simulink model "birotorPVTOL"  (Simulink 7.5)
settings: Solver=ode45  StartTime=0.0  StopTime=10  RelTol=1e-3
values from neighbouring files (symbols this model uses):
  x0 = input('Introduzca x0: ')    [practicaCuadriRotor.m]    (also in practicaPVTOL.m)
  xf = input('Introduzca xf: ')    [practicaCuadriRotor.m]    (also in practicaPVTOL.m)
  y0 = input('Introduzca y0: ')    [practicaCuadriRotor.m]    (also in practicaPVTOL.m)
  yf = input('Introduzca yf: ')    [practicaCuadriRotor.m]    (also in practicaPVTOL.m)
settings Model: Creator=Celeste Anaid  LastModifiedBy=Mariano
settings OptimizationCC: ExpressionDepthLimit=128
settings DebuggingCC: MultiTaskDSMMsg=warning  MultiTaskCondExecSysMsg=none  FcnCallInpInsideContextMsg=Enable All  StrictBusMsg=None
settings RTWCC: IncludeERTFirstTime=on
settings CodeAppCC: CustomSymbolStrType=$N$R$M_T
settings GRTTargetCC: CombineOutputUpdateFcns=on

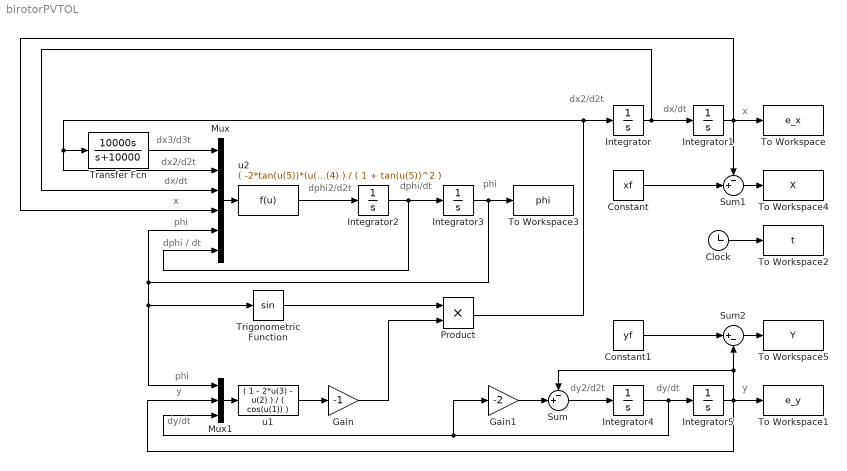
== system birotorPVTOL ==
  note: dy/dt
  note: y
  note: phi
  note: dy/dt
  note: dy2/d2t
  note: phi
  note: dphi/dt
  note: dphi2/d2t
  note: phi
  note: dphi / dt
  note: x
  note: dx/dt
  note: dx3/d3t
  note: dx2/d2t
  note: x
  note: dx/dt
  note: dx2/d2t
  note: y
  Clock : Clock
      settings: Decimation=10
  Constant : Constant  Value=xf  OutDataType=fixdt(1, 16)  OutScaling=2^0
  Constant1 : Constant  Value=yf  OutDataType=fixdt(1, 16)  OutScaling=2^0
  Gain : Gain  Gain=-1
  Gain1 : Gain  Gain=-2
  Integrator{,2..4} (4 alike) : Integrator
  Integrator1 : Integrator  InitialCondition=xf-x0
  Integrator5 : Integrator  InitialCondition=yf-y0
  Mux : Mux  Inputs=6
  Mux1 : Mux  Inputs=3
  Product : Product
  Sum : Sum  Inputs=-+|
  Sum1 : Sum  Inputs=-+|  OutDataType=fixdt(1, 16)  OutScaling=2^0
  Sum2 : Sum  Inputs=|+-  OutDataType=fixdt(1, 16)  OutScaling=2^0
  To Workspace : ToWorkspace  VariableName=e_x  SampleTime=-1  SaveFormat=Array
  To Workspace1 : ToWorkspace  VariableName=e_y  SampleTime=-1  SaveFormat=Array
  To Workspace2 : ToWorkspace  VariableName=t  SampleTime=-1  SaveFormat=Array
  To Workspace3 : ToWorkspace  VariableName=phi  SampleTime=-1  SaveFormat=Array
  To Workspace4 : ToWorkspace  VariableName=X  SampleTime=-1  SaveFormat=Array
  To Workspace5 : ToWorkspace  VariableName=Y  SampleTime=-1  SaveFormat=Array
  Transfer Fcn : TransferFcn  Numerator=[10000 0]  Denominator=[1 10000]
  Trigonometric Function : Trigonometry
  u1 : Fcn  Expr=( 1 - 2*u(3) - u(2) ) / ( cos(u(1)) )
  u2 : Fcn  Expr=|
      | ( -2*tan(u(5))*(u(6)^2)*(1+tan(u(5))^2)
      | -2*(1+tan(u(5))^2)*u(6) -tan(u(5)) +2*u(1) +5*u(2) +4*u(3) + u(4) ) / ( 1 + tan(u(5))^2 )
  wires:
  Transfer Fcn/1 -> Mux/1
  Integrator/1 -> Mux/3, Integrator1/1
  Integrator1/1 -> Mux/4, To Workspace/1, Sum1/1
  Mux/1 -> u2/1
  u2/1 -> Integrator2/1
  Integrator2/1 -> Integrator3/1, Mux/6
  Integrator3/1 -> To Workspace3/1, Mux/5, Mux1/1, Trigonometric Function/1
  Sum/1 -> Integrator4/1
  Mux1/1 -> u1/1
  Integrator5/1 -> To Workspace1/1, Mux1/2, Sum/1, Sum2/2
  Clock/1 -> To Workspace2/1
  Integrator4/1 -> Integrator5/1, Gain1/1, Mux1/3
  Gain1/1 -> Sum/2
  Trigonometric Function/1 -> Product/1
  u1/1 -> Gain/1
  Gain/1 -> Product/2
  Product/1 -> Integrator/1, Transfer Fcn/1, Mux/2
  Sum1/1 -> To Workspace4/1
  Constant/1 -> Sum1/2
  Sum2/1 -> To Workspace5/1
  Constant1/1 -> Sum2/1
